simulink model "IMU_UKF_circle_exp_sampling_rate_issue"  (R2025a)
settings: Solver=FixedStepAuto  StartTime=0.0  StopTime=inf  FixedStep=0.01  RelTol=1e-3
undefined symbols (not defined in the file or in its folder): National_Instruments, PCI
libraries: sldrtlib x3, slpidlib x2, hostiolib x1
settings Model: Creator=dperera  LastModifiedBy=dperera

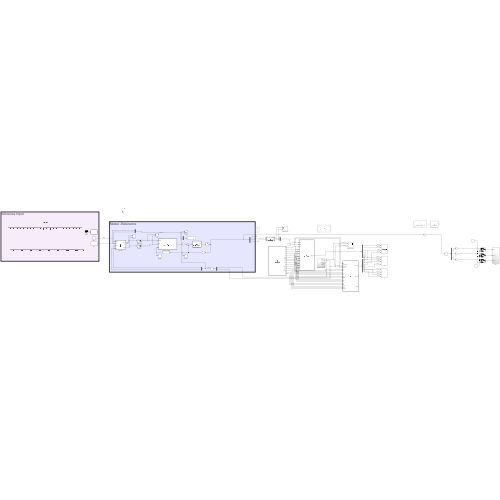
[thumbnail: Simulink's stored preview of the top-level diagram]
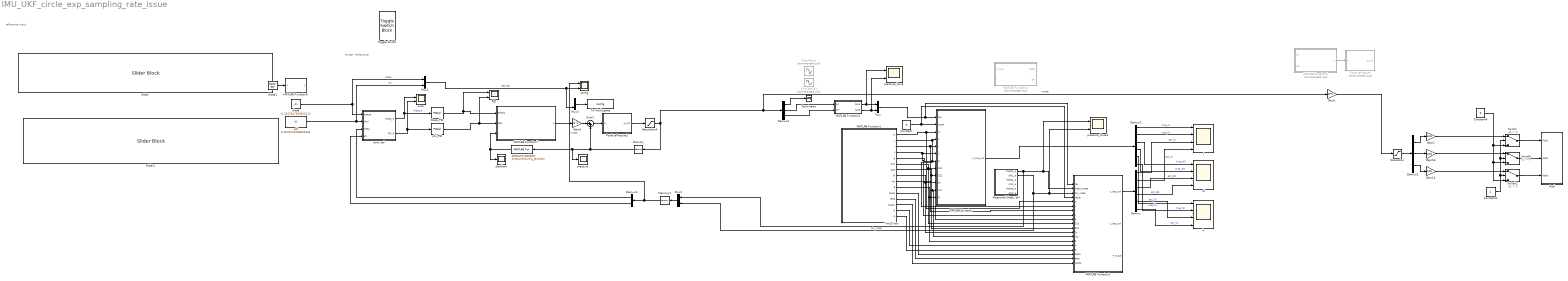
== system IMU_UKF_circle_exp_sampling_rate_issue ==
  note: reference Input
  note: Model -Reference
  Constant : Constant  Value=0
  Constant1 : Constant
  Constant4 : Constant  Value=0
  Demux : Demux  Outputs=6
  Demux1 : Demux  Outputs=6
  Demux2 : Demux  Outputs=3
  Demux3 : Demux  Outputs=2
  Demux4 : Demux  Outputs=3
  Gain1 : Gain  Gain=1e-5
  Gain14 : Gain  Gain=10/9
  Gain16 : Gain  Gain=10/9
  Gain2 : Gain  Gain=10/9
  Gain3 : Gain  Gain=0.1
  Jacobian : Scope
      settings: ActiveDisplayYMinimum=-10.825317547305481  ActiveDisplayYMaximum=10.825317547305481  DataLoggingVariableName=ScopeData5
  MATLAB Function : MATLAB Function  TreatAsAtomicUnit=on
  MATLAB Function1 : MATLAB Function  TreatAsAtomicUnit=on
  MATLAB Function2 : MATLAB Function  Commented=on  TreatAsAtomicUnit=on
  MATLAB Function3 : MATLAB Function  TreatAsAtomicUnit=on
  MATLAB Function4 : MATLAB Function  TreatAsAtomicUnit=on
  MATLAB Function5 : MATLAB Function  Commented=on  TreatAsAtomicUnit=on
  MATLAB Function6 : MATLAB Function  TreatAsAtomicUnit=on
  MATLAB Function7 : MATLAB Function  TreatAsAtomicUnit=on
  "Measured theta, phi" : Subsystem
  Memory : Memory  InitialCondition=[1; 1.1; 1]  LinearizeMemory=on  LinearizeAsDelay=on
  Memory1 : Memory  InitialCondition=[0.0001, 0.0001]  LinearizeMemory=on  LinearizeAsDelay=on
  Mux{,1..3} (4 alike) : Mux  Inputs=2
  PID : Scope  NumInputPorts=2
      settings: ActiveDisplayYMinimum=-3.9804584732791981  ActiveDisplayYMaximum=3.8453740981888478  DataLoggingVariableName=ScopeData6
  PositivePresure : MATLAB Function  Commented=on  TreatAsAtomicUnit=on
  PositivePresure1 : MATLAB Function  TreatAsAtomicUnit=on
  "Red " : Subsystem
  Saturation : Saturate  UpperLimit=3  LowerLimit=0
  Saturation4 : Saturate  UpperLimit=300000  LowerLimit=0
  Sine Wave : Sin  Commented=on  Amplitude=2.5e4  Frequency=0.5  SampleTime=0
  Sine Wave1 : Sin  Commented=on  Amplitude=2.5e4  Frequency=0.5  SampleTime=0
  Slider : SliderBlock  ScaleMin=-3.14  ScaleMax=3.14
  Slider1 : SliderBlock  ScaleMax=3.14
  Sum2 : Sum  Inputs=|++
  Switch : Switch  Criteria=u2 > Threshold  SaturateOnIntegerOverflow=off  InputSameDT=off
  Switch1 : Switch  Criteria=u2 > Threshold  SaturateOnIntegerOverflow=off  InputSameDT=off
  Switch2 : Switch  Criteria=u2 > Threshold  SaturateOnIntegerOverflow=off  InputSameDT=off
  Terminator : Terminator
  To Workspace : ToWorkspace  VariableName=config  SaveFormat=Structure With Time  SampleTime=-1
  Toggle Switch : ToggleSwitchBlock
  config : Scope  NumInputPorts=2
      settings: ActiveDisplayYMinimum=-3.926205418823844  ActiveDisplayYMaximum=3.9199222335166648  DataLoggingVariableName=ScopeData7
  dl : Scope  NumInputPorts=4
      settings: ActiveDisplayYMinimum=-0.11562375107326617  ActiveDisplayYMaximum=0.16522740194349217
  error : Scope  NumInputPorts=2
      settings: ActiveDisplayYMinimum=-1.7062614665873941  ActiveDisplayYMaximum=3.7647403361072445  DataLoggingVariableName=ScopeData9
  error cal : MATLAB Function  TreatAsAtomicUnit=on
  h : Scope  NumInputPorts=4
      settings: ActiveDisplayYMinimum=-3.6910086116177509E-9  ActiveDisplayYMaximum=1.6868676985022998E-9  DataLoggingVariableName=ScopeData2
  l : Scope  NumInputPorts=4
      settings: ActiveDisplayYMinimum=-0.05861032867923114  ActiveDisplayYMaximum=0.027492958113080231
  phi : Constant  Value=0.4033234086825366
  phi_PID : slpidlib/PID Controller  Controller=PID  Form=Parallel  TimeDomain=Continuous-time  UseExternalTs=off  SampleTime=-1  IntegratorMethod=Forward Euler  FilterMethod=Forward Euler  ControllerParametersSource=internal  P=0.1  I=0.01  UseKiTs=off  D=0.00001  UseExternalDerivativeSource=off  N=100  UseFilter=on  TunerSelectOption=Transfer Function Based (PID Tuner App)  InitialConditionSource=internal  InitialConditionForIntegrator=0  InitialConditionForFilter=0  DifferentiatorICPrevScaledInput=0  ExternalReset=none  TrackingMode=off  Kt=1  LimitOutput=on  SatLimitsSource=internal  UpperSaturationLimit=inf  LowerSaturationLimit=-inf  LinearizeAsGain=off  AntiWindupMode=back-calculation  Kb=1  LimitIntegrator=off  UpperIntegratorSaturationLimit=10  LowerIntegratorSaturationLimit=-10  POutMin=[]  POutMax=[]  IOutMin=[]  IOutMax=[]  DOutMin=[]  DOutMax=[]  NOutMin=[]  NOutMax=[]  SumOutMin=[]  SumOutMax=[]  SaturationOutMin=[]  SaturationOutMax=[]  PParamMin=[]  PParamMax=[]  IParamMin=[]  IParamMax=[]  DParamMin=[]  DParamMax=[]  NParamMin=[]  NParamMax=[]  KbParamMin=[]  KbParamMax=[]  KtParamMin=[]  KtParamMax=[]  KbOutMin=[]  KbOutMax=[]  KtOutMin=[]  KtOutMax=[]  IntegratorOutMin=[]  IntegratorOutMax=[]  FilterOutMin=[]  FilterOutMax=[]  SumI1OutMin=[]  SumI1OutMax=[]  SumI2OutMin=[]  SumI2OutMax=[]  SumI3OutMin=[]  SumI3OutMax=[]  SumI4OutMin=[]  SumI4OutMax=[]  SumDOutMin=[]  SumDOutMax=[]  DifferentiatorOutMin=[]  DifferentiatorOutMax=[]  FilterDiffOutCoefMin=[]  FilterDiffOutCoefMax=[]  ReciprocalOutMin=[]  ReciprocalOutMax=[]  SumDenOutMin=[]  SumDenOutMax=[]  SumNumOutMin=[]  SumNumOutMax=[]  DivideOutMin=[]  DivideOutMax=[]  UdiffTsProdOutMin=[]  UdiffTsProdOutMax=[]  NTsProdOutMin=[]  NTsProdOutMax=[]  UintegralTsProdOutMin=[]  UintegralTsProdOutMax=[]  UngainTsProdOutMin=[]  UngainTsProdOutMax=[]  ClampingZeroOutDataTypeStr=Inherit: Inherit via back propagation  ClampingZeroOutMin=[]  ClampingZeroOutMax=[]  FilterDenConstantOutDataTypeStr=Inherit: Inherit via back propagation  FilterDenConstantOutMin=[]  FilterDenConstantOutMax=[]  PCopyOutDataTypeStr=Inherit: Inherit via back propagation  PCopyOutMin=[]  PCopyOutMax=[]  NCopyOutDataTypeStr=Inherit: Inherit via back propagation  NCopyOutMin=[]  NCopyOutMax=[]  IntegratorContinuousStateAttributes=''  IntegratorStateMustResolveToSignalObject=off  IntegratorRTWStateStorageClass=Auto  FilterContinuousStateAttributes=''  FilterStateMustResolveToSignalObject=off  FilterRTWStateStorageClass=Auto  ParallelPVariant=InternalParameters  IdealPVariant=Disabled  IVariant=InternalParameters  DVariant=InternalParameters  IntegratorVariant=Continuous  SatVariant=Enabled  AWVariant=BackCalculation  PCopyVariant=Disabled  TRVariant=Disabled  FdbkBlocksVariant=Forward  IdealPFdbkVariant=Disabled  SatFdbkVariant=Disabled  DerivativeFilterVariant=ContFilter  NVariant=InternalParameters  NCopyVariant=Disabled  FilterICVariant=InternalICsFilter  IntegratorICVariant=InternalICs  ExternalResetVariant=Disabled  TRSumVariant=Passthrough  SumFdbkVariant=Disabled  SumVariant=Sum_PID  TsampFilterVariant=InternalTs  TsampNgainVariant=Passthrough  TsampIntegralVariant=Disabled_SignalSpec  ExternalSaturationOutDataTypeStr=Inherit: Same as second input  DerivativeSourceVariant=ErrorSignal  PreIntVariant=InternalPreInt
  pressure : Scope
      settings: ActiveDisplayYMinimum=-37499.999999999993  ActiveDisplayYMaximum=337500  DataLoggingVariableName=ScopeData10
  pressure_force : Scope  NumInputPorts=2
      settings: ActiveDisplayYMinimum=-1  ActiveDisplayYMaximum=1  DataLoggingVariableName=ScopeData3
  pressure_force1 : Scope  NumInputPorts=2
      settings: ActiveDisplayYMinimum=-0.05267150170136882  ActiveDisplayYMaximum=1.3490874232227761  DataLoggingVariableName=ScopeData4
  pressure_jacobian : MATLABFcn  MATLABFcn=pressure2config_Jacobian  OutputDimensions=[2 3]  OutputSignalType=real  Output1D=off
  theta : Constant  Value=-0.2347847506630112
  theta1 : SignalGenerator  WaveForm=sawtooth  Amplitude=pi  Frequency=0.2*2*pi  Units=rad/sec  VectorParams1D=off
  theta_PID : slpidlib/PID Controller  Controller=PID  Form=Parallel  TimeDomain=Continuous-time  UseExternalTs=off  SampleTime=-1  IntegratorMethod=Forward Euler  FilterMethod=Forward Euler  ControllerParametersSource=internal  P=0.1  I=0.01  UseKiTs=off  D=0.0001  UseExternalDerivativeSource=off  N=100  UseFilter=on  TunerSelectOption=Transfer Function Based (PID Tuner App)  InitialConditionSource=internal  InitialConditionForIntegrator=0  InitialConditionForFilter=0  DifferentiatorICPrevScaledInput=0  ExternalReset=none  TrackingMode=off  Kt=1  LimitOutput=on  SatLimitsSource=internal  UpperSaturationLimit=inf  LowerSaturationLimit=-inf  LinearizeAsGain=off  AntiWindupMode=back-calculation  Kb=1  LimitIntegrator=off  UpperIntegratorSaturationLimit=10  LowerIntegratorSaturationLimit=-10  POutMin=[]  POutMax=[]  IOutMin=[]  IOutMax=[]  DOutMin=[]  DOutMax=[]  NOutMin=[]  NOutMax=[]  SumOutMin=[]  SumOutMax=[]  SaturationOutMin=[]  SaturationOutMax=[]  PParamMin=[]  PParamMax=[]  IParamMin=[]  IParamMax=[]  DParamMin=[]  DParamMax=[]  NParamMin=[]  NParamMax=[]  KbParamMin=[]  KbParamMax=[]  KtParamMin=[]  KtParamMax=[]  KbOutMin=[]  KbOutMax=[]  KtOutMin=[]  KtOutMax=[]  IntegratorOutMin=[]  IntegratorOutMax=[]  FilterOutMin=[]  FilterOutMax=[]  SumI1OutMin=[]  SumI1OutMax=[]  SumI2OutMin=[]  SumI2OutMax=[]  SumI3OutMin=[]  SumI3OutMax=[]  SumI4OutMin=[]  SumI4OutMax=[]  SumDOutMin=[]  SumDOutMax=[]  DifferentiatorOutMin=[]  DifferentiatorOutMax=[]  FilterDiffOutCoefMin=[]  FilterDiffOutCoefMax=[]  ReciprocalOutMin=[]  ReciprocalOutMax=[]  SumDenOutMin=[]  SumDenOutMax=[]  SumNumOutMin=[]  SumNumOutMax=[]  DivideOutMin=[]  DivideOutMax=[]  UdiffTsProdOutMin=[]  UdiffTsProdOutMax=[]  NTsProdOutMin=[]  NTsProdOutMax=[]  UintegralTsProdOutMin=[]  UintegralTsProdOutMax=[]  UngainTsProdOutMin=[]  UngainTsProdOutMax=[]  ClampingZeroOutDataTypeStr=Inherit: Inherit via back propagation  ClampingZeroOutMin=[]  ClampingZeroOutMax=[]  FilterDenConstantOutDataTypeStr=Inherit: Inherit via back propagation  FilterDenConstantOutMin=[]  FilterDenConstantOutMax=[]  PCopyOutDataTypeStr=Inherit: Inherit via back propagation  PCopyOutMin=[]  PCopyOutMax=[]  NCopyOutDataTypeStr=Inherit: Inherit via back propagation  NCopyOutMin=[]  NCopyOutMax=[]  IntegratorContinuousStateAttributes=''  IntegratorStateMustResolveToSignalObject=off  IntegratorRTWStateStorageClass=Auto  FilterContinuousStateAttributes=''  FilterStateMustResolveToSignalObject=off  FilterRTWStateStorageClass=Auto  ParallelPVariant=InternalParameters  IdealPVariant=Disabled  IVariant=InternalParameters  DVariant=InternalParameters  IntegratorVariant=Continuous  SatVariant=Enabled  AWVariant=BackCalculation  PCopyVariant=Disabled  TRVariant=Disabled  FdbkBlocksVariant=Forward  IdealPFdbkVariant=Disabled  SatFdbkVariant=Disabled  DerivativeFilterVariant=ContFilter  NVariant=InternalParameters  NCopyVariant=Disabled  FilterICVariant=InternalICsFilter  IntegratorICVariant=InternalICs  ExternalResetVariant=Disabled  TRSumVariant=Passthrough  SumFdbkVariant=Disabled  SumVariant=Sum_PID  TsampFilterVariant=InternalTs  TsampNgainVariant=Passthrough  TsampIntegralVariant=Disabled_SignalSpec  ExternalSaturationOutDataTypeStr=Inherit: Same as second input  DerivativeSourceVariant=ErrorSignal  PreIntVariant=InternalPreInt
  wires:
  MATLAB Function1/1(m) -> MATLAB Function3/5(m), MATLAB Function/3(m)
  MATLAB Function1/2(L) -> MATLAB Function/4(L), MATLAB Function3/6(L)
  MATLAB Function1/3(r) -> MATLAB Function3/7(r), MATLAB Function/5(r)
  MATLAB Function1/4(k) -> MATLAB Function3/8(k), MATLAB Function/6(k)
  MATLAB Function1/5(g) -> MATLAB Function3/9(g), MATLAB Function/7(g)
  MATLAB Function1/6(D11) -> MATLAB Function3/10(D11), MATLAB Function/8(D11)
  MATLAB Function1/7(D22) -> MATLAB Function3/11(D22), MATLAB Function/9(D22)
  MATLAB Function1/8(Ts) -> MATLAB Function3/12(Ts), MATLAB Function/10(Ts)
  MATLAB Function1/9(rho) -> MATLAB Function3/13(rho), MATLAB Function/11(rho)
  MATLAB Function1/10(B) -> MATLAB Function3/14(B), MATLAB Function/12(B)
  MATLAB Function/1(x_true_out) -> Demux1/1
  MATLAB Function1/11(alpha) -> MATLAB Function3/17(alpha)
  MATLAB Function1/12(beta) -> MATLAB Function3/18(beta)
  MATLAB Function1/13(kappa) -> MATLAB Function3/19(kappa)
  MATLAB Function1/14(Q) -> MATLAB Function3/15(Q)
  MATLAB Function1/15(R) -> MATLAB Function3/16(R)
  Constant/1 -> MATLAB Function3/4(reset), MATLAB Function/2(reset)
  Mux/1 -> MATLAB Function3/1(tau), MATLAB Function/1(tau)
  MATLAB Function3/1(x_hat_out) -> Demux/1
  Demux1/1 -> l/1  "true_l2"
  Demux/1 -> l/3  "est_l2"
  Demux1/2 -> l/2  "true_l3"
  Demux/2 -> l/4  "est_l3"
  Demux1/3 -> dl/1  "true_dl2"
  Demux1/4 -> dl/2  "true_dl3"
  Demux/3 -> dl/3  "est_dl2"
  Demux/4 -> dl/4  "est_dl3"
  Demux1/5 -> h/1  "true_h1"
  Demux1/6 -> h/2  "true_h2"
  Demux/5 -> h/3  "est_h1"
  Demux/6 -> h/4  "est_h2"
  MATLAB Function4/1(tau2) -> pressure_force/1, Mux/1
  MATLAB Function4/2(tau3) -> Mux/2, pressure_force/2
  Demux4/2 -> MATLAB Function4/1(p2)
  Demux4/3 -> MATLAB Function4/2(p3)
  "Measured theta, phi"/1(theta1_a) -> Mux2/1, pressure_force1/1, MATLAB Function3/2(theta_meas)  "theta_meas"
  "Measured theta, phi"/2(phi1_a) -> Mux2/2, pressure_force1/2, MATLAB Function3/3(phi_meas)  "phi_meas"
  Demux2/2 -> Gain16/1
  Demux2/3 -> Gain14/1
  Switch2/1 -> "Red "/3(Red3)
  Constant4/1 -> Switch2/3, Switch1/3, Switch/3
  Demux2/1 -> Gain2/1
  Gain16/1 -> Switch1/1
  Gain2/1 -> Switch/1
  Switch1/1 -> "Red "/2(Red2)
  Switch/1 -> "Red "/1(Red1)
  MATLAB Function5/1(p) -> PositivePresure/1(p)
  Gain14/1 -> Switch2/1
  Saturation/1 -> Demux2/1
  Constant1/1 -> Switch2/2, Switch1/2, Switch/2
  Mux3/1 -> To Workspace/1
  error cal/2(phi_e) -> error/2, phi_PID/1
  Mux1/1 -> config/2, Mux3/2  "desired"
  theta/1 -> Mux1/1, error cal/1(thetad)  "theta"
  phi/1 -> Mux1/2, error cal/2(phid)  "phi"
  Sum2/1 -> PositivePresure1/1(p)
  phi_PID/1 -> PID/2, MATLAB Function7/2(dphi)
  Demux3/2 -> error cal/4(phi)
  theta1/1 -> MATLAB Function6/1(u)
  PositivePresure1/1(p_out) -> Saturation4/1
  Gain3/1 -> Sum2/1
  Memory1/1 -> config/1, Demux3/1  "model"
  pressure_jacobian/1 -> Jacobian/1, MATLAB Function7/3(J)
  MATLAB Function7/1(p) -> Gain3/1
  Memory/1 -> pressure/1, pressure_jacobian/1, Sum2/2
  Saturation4/1 -> Gain1/1, Demux4/1, Memory/1  "model"
  Demux3/1 -> error cal/3(theta)
  error cal/1(theta_e) -> error/1, theta_PID/1  "theta_e"
  theta_PID/1 -> PID/1, MATLAB Function7/1(dtheta)
  Mux2/1 -> Memory1/1
  Gain1/1 -> Saturation/1
  Demux4/1 -> Terminator/1

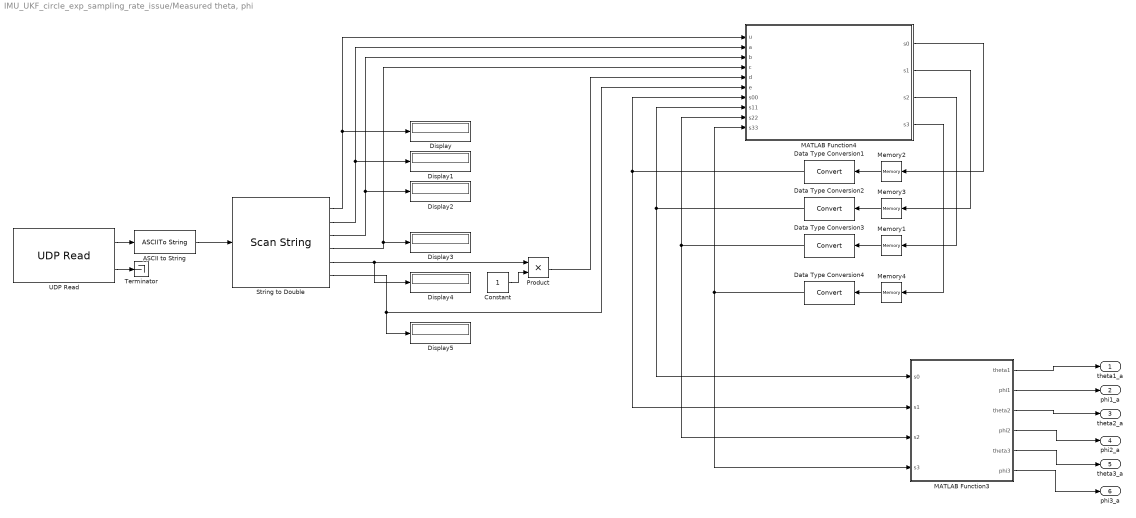
== system IMU_UKF_circle_exp_sampling_rate_issue/Measured theta, phi ==
  ASCII to String : ASCIIToString
  Constant : Constant
  Data Type Conversion{1..4} (4 alike) : DataTypeConversion  SaturateOnIntegerOverflow=off  RndMeth=Floor
  Display{,1..5} (6 alike) : Display
  MATLAB Function3 : MATLAB Function  TreatAsAtomicUnit=on
  MATLAB Function4 : MATLAB Function  TreatAsAtomicUnit=on
  Memory1 : Memory  InitialCondition=[1.0,0,0,0,0,1]  InheritSampleTime=on
  Memory2 : Memory  InitialCondition=[0.0,0,0,0,0,1]  InheritSampleTime=on
  Memory3 : Memory  InitialCondition=[1.0,0,0,0,0,1]  InheritSampleTime=on
  Memory4 : Memory  InitialCondition=[1.0,0,0,0,0,1]  InheritSampleTime=on
  Product : Product
  String to Double : ScanString  Format="\"%f %f %f %f %f %f\""
  Terminator : Terminator
  UDP Read : hostiolib/UDP Read  localURL='0.0.0.0'  localPort=60002  remoteURL='localhost'  remotePort=-1  recvBufferSize=1024  dims=255  signalDatatype=uint8  isVarSize=off  showBlockingTime=on  blockingTime=0  sampletime=0.01  blockPlatform=HOST  hoistedMaskSrc=UDP Read/UDP Read Sim/UDP Read
  theta1_a : Outport
  phi1_a : Outport  Port=2
  theta2_a : Outport  Port=3
  phi2_a : Outport  Port=4
  theta3_a : Outport  Port=5
  phi3_a : Outport  Port=6
  wires:
  ASCII to String/1 -> String to Double/1
  Memory4/1 -> Data Type Conversion4/1
  Constant/1 -> Product/2
  UDP Read/2 -> Terminator/1
  UDP Read/1 -> ASCII to String/1
  String to Double/2 -> MATLAB Function4/2(a), Display1/1
  String to Double/1 -> Display/1, MATLAB Function4/1(u)
  MATLAB Function4/3(s2) -> Memory1/1
  Data Type Conversion4/1 -> MATLAB Function3/4(s3), MATLAB Function4/10(s33)
  String to Double/6 -> Display5/1, MATLAB Function4/6(e)
  Product/1 -> MATLAB Function4/5(d)
  String to Double/4 -> MATLAB Function4/4(c), Display3/1
  String to Double/5 -> Display4/1, Product/1
  Memory2/1 -> Data Type Conversion1/1
  Data Type Conversion2/1 -> MATLAB Function3/1(s0), MATLAB Function4/8(s11)
  Memory1/1 -> Data Type Conversion3/1
  MATLAB Function4/4(s3) -> Memory4/1
  MATLAB Function4/2(s1) -> Memory3/1
  Data Type Conversion3/1 -> MATLAB Function3/3(s2), MATLAB Function4/9(s22)
  Memory3/1 -> Data Type Conversion2/1
  MATLAB Function4/1(s0) -> Memory2/1
  Data Type Conversion1/1 -> MATLAB Function3/2(s1), MATLAB Function4/7(s00)
  String to Double/3 -> MATLAB Function4/3(b), Display2/1
  MATLAB Function3/1(theta1) -> theta1_a/1
  MATLAB Function3/2(phi1) -> phi1_a/1
  MATLAB Function3/3(theta2) -> theta2_a/1
  MATLAB Function3/4(phi2) -> phi2_a/1
  MATLAB Function3/5(theta3) -> theta3_a/1
  MATLAB Function3/6(phi3) -> phi3_a/1

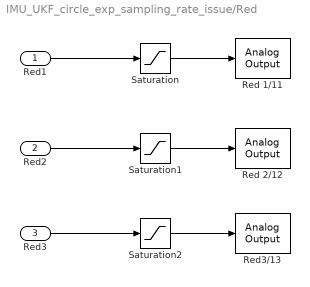
== system IMU_UKF_circle_exp_sampling_rate_issue/Red  ==
  Red1 : Inport
  Red2 : Inport  Port=2
  Red3 : Inport  Port=3
  Red 1/11 : sldrtlib/Analog Output  SampleTime=0.01  MaxMissedTicks=inf  ShowMissedTicks=off  YieldWhenWaiting=on  DrvName=National_Instruments/PCI-6703  DrvAddress=4294967295  DrvOptions=0  Channels=1  RangeMode=1  VoltRange=1  InitialValue=0  FinalValue=0
      settings: AttributesFormatString=National Instruments\nPCI-6703 [auto]
  Red 2/12 : sldrtlib/Analog Output  SampleTime=0.01  MaxMissedTicks=inf  ShowMissedTicks=off  YieldWhenWaiting=on  DrvName=National_Instruments/PCI-6703  DrvAddress=4294967295  DrvOptions=0  Channels=2  RangeMode=1  VoltRange=1  InitialValue=0  FinalValue=0
      settings: AttributesFormatString=National Instruments\nPCI-6703 [auto]
  Red3/13 : sldrtlib/Analog Output  SampleTime=0.01  MaxMissedTicks=inf  ShowMissedTicks=off  YieldWhenWaiting=on  DrvName=National_Instruments/PCI-6703  DrvAddress=4294967295  DrvOptions=0  Channels=3  RangeMode=1  VoltRange=1  InitialValue=0  FinalValue=0
      settings: AttributesFormatString=National Instruments\nPCI-6703 [auto]
  Saturation : Saturate  UpperLimit=7  LowerLimit=0
  Saturation1 : Saturate  UpperLimit=7  LowerLimit=0
  Saturation2 : Saturate  UpperLimit=7  LowerLimit=0
  wires:
  Red1/1 -> Saturation/1
  Saturation/1 -> Red 1/11/1
  Saturation1/1 -> Red 2/12/1
  Saturation2/1 -> Red3/13/1
  Red2/1 -> Saturation1/1
  Red3/1 -> Saturation2/1

== matlab function IMU_UKF_circle_exp_sampling_rate_issue/MATLAB Function4 ==
  data: tau2 output; tau3 output; p2 input; p3 input
function [tau2,tau3] = pressures(p2, p3)
%#codegen

A = pi * (0.013/2)^2;
tau2 = p2*A;
tau3 = p3*A;

end

== matlab function IMU_UKF_circle_exp_sampling_rate_issue/Measured theta, phi/MATLAB Function3 ==
  data: s0 input; theta1 output; s1 input; phi1 output; s2 input; s3 input; theta2 output; phi2 output; theta3 output; phi3 output
function [theta1,phi1,theta2,phi2,theta3,phi3]= fcn(s0,s1,s2,s3)

s0_start=[0,0,0,1];
s1_start=[0,0,0,1];
s2_start=[0,0,0,1];
s3_start=[0,0,0,1];


%base=[base1(3),base1(4),base1(5),base1(6)];

sensor0=[s0(6),s0(3),s0(5),s0(4)]; %base
sensor1=[s1(6),s1(3),s1(5),s1(4)];
sensor2=[s2(6),s2(3),s2(5),s2(4)];
sensor3=[s3(6),s3(3),s3(5),s3(4)];

%tip_relative_base=quatmultiply(quatmultiply(tip,quatinv(tip_start)),quatinv(quatmultiply(base,quatinv(base_start))));

sensor1_relative_sensor0=quatmultiply(quatmultiply(sensor1,quatinv(s1_start)),quatinv(quatmultiply(sensor0,quatinv(s0_start))));
sensor2_relative_sensor1=quatmultiply(quatmultiply(sensor2,quatinv(s2_start)),quatinv(quatmultiply(sensor1,quatinv(s1_start))));
sensor3_relative_sensor2=quatmultiply(quatmultiply(sensor3,quatinv(s3_start)),quatinv(quatmultiply(sensor2,quatinv(s2_start))));

%rotMat = quat2tform(tip_relative_base);
rotMat1 = quat2tform(sensor1_relative_sensor0); % only base
theta1= (atan2(rotMat1(2,3),rotMat1(1,3)));
phi1= (acos(rotMat1(3,3)));

rotMat2 = quat2tform(sensor2_relative_sensor1); 
theta2=  (atan2(rotMat2(2,3),rotMat2(1,3)));
phi2= (acos(rotMat2(3,3)));

rotMat3 = quat2tform(sensor3_relative_sensor2); 
theta3= (atan2(rotMat3(2,3),rotMat3(1,3)));
phi3= (acos(rotMat3(3,3)));


end

== matlab function IMU_UKF_circle_exp_sampling_rate_issue/Measured theta, phi/MATLAB Function4 ==
  data: u input; s0 output; a input; b input; c input; d input; e input; s00 input; s11 input; s1 output; s22 input; s33 input; s2 output; s3 output
function [s0,s1,s2,s3]= fcn(u,a,b,c,d,e,s00,s11,s22,s33)
if u==1.0
    %base1=[double(u),double(a),double(b),double(c),double(d),double(e)];
    s00(1)=double(u);
    s00(2)=double(a);
    s00(3)=double(b); %x
    s00(4)=double(c); %y
    s00(5)=double(d); %z
    s00(6)=double(e); %w

elseif u==2.0
    %tip1=[double(u),double(a),double(b),double(c),double(d),double(e)];
    s11(1)=double(u);
    s11(2)=double(a);
    s11(3)=double(b);
    s11(4)=double(c);
    s11(5)=double(d);
    s11(6)=double(e);
elseif u==3.0
    %tip1=[double(u),double(a),double(b),double(c),double(d),double(e)];
    s22(1)=double(u);
    s22(2)=double(a);
    s22(3)=double(b);
    s22(4)=double(c);
    s22(5)=double(d);
    s22(6)=double(e);
elseif u==4.0
    %tip1=[double(u),double(a),double(b),double(c),double(d),double(e)];
    s33(1)=double(u);
    s33(2)=double(a);
    s33(3)=double(b);
    s33(4)=double(c);
    s33(5)=double(d);
    s33(6)=double(e);
end
    s0=s00;
    s1=s11;
    s2=s22;
    s3=s33;

end

== matlab function IMU_UKF_circle_exp_sampling_rate_issue/MATLAB Function5 ==
  data: p2 input; p output; p3 input
function p = Measurement_Block(p2, p3)
%#codegen

p = [-(p2+p3); p2; p3];

end

== matlab function IMU_UKF_circle_exp_sampling_rate_issue/PositivePresure ==
  data: p input; p_out output
function p_out  = PositivePressure(p)

    minP = min(p);
    maxP = max(p);
    
    p_pos = p-minP;
    % p_pos_norm = p_pos / (maxP - minP) * maxP; % Normalize the positive pressures
    
    p_out = p_pos/max(p_pos) * maxP;
    
end

== matlab function IMU_UKF_circle_exp_sampling_rate_issue/MATLAB Function6 ==
  data: u input; y output
function y = fcn(u)

y = wrapToPi(u - pi);

== matlab function IMU_UKF_circle_exp_sampling_rate_issue/MATLAB Function7 ==
  data: dtheta input; p output; dphi input; J input
function p  = config3pressure_projection(dtheta, dphi, J)

    p = J \ [dtheta; dphi];
end

== matlab function IMU_UKF_circle_exp_sampling_rate_issue/PositivePresure1 ==
  data: p input; p_out output
function p_out  = PositivePressure(p)

    minP = min(p);
    maxP = max(p);
    
    p_pos = p-minP;
    % p_pos_norm = p_pos / (maxP - minP) * maxP; % Normalize the positive pressures
    
    p_out = p_pos/max(p_pos) * maxP;
    
end

== matlab function IMU_UKF_circle_exp_sampling_rate_issue/error cal ==
  data: thetad input; theta_e output; phid input; theta input; phi input; phi_e output
function [theta_e, phi_e]    = fcn(thetad, phid, theta, phi)

    % qd = [thetad;phid];
    % q = [theta;phi];
    % 
    % abs_diff = abs(thetad-theta);
    % abs_diff_mod = abs(mod(thetad, 2*pi)-mod(theta, 2*pi));
    % 
    % if abs_diff < abs_diff_mod
    %     error = qd-q;
    % else
    %     error = mod(qd, 2*pi) - mod(q,2*pi);
    % end
    % 
    % if error(1) < 0.0001
    %     error(1) = 0;
    % end
    % 
    % if error(2) < 0.0001
    %     error(2) = 0;
    % end
    % 
    % theta_e = error(1);
    % phi_e = error(2);

        % Compute signed angular differences in (-pi, pi]
    theta_e = atan2(sin(thetad - theta), cos(thetad - theta));
    phi_e   = atan2(sin(phid - phi), cos(phid - phi));

    % Optional: zero small errors
    if abs(theta_e) < 1e-4
        theta_e = 0;
    end
    if abs(phi_e) < 1e-4
        phi_e = 0;
    end

end

== matlab function IMU_UKF_circle_exp_sampling_rate_issue/MATLAB Function1 ==
  data: m output; L output; r output; k output; g output; D11 output; D22 output; Ts output; rho output; B output; alpha output; beta output; kappa output; Q output; R output
function [m, L, r, k, g, D11, D22, Ts, rho, B, alpha, beta, kappa, Q, R] = parameters()
%#codegen

m    = 0.10;
L    = [0.0; 0.278; 0.0];
r    = 0.013;
k    = [0.0; 2.4e3; 2.4e3];
g    = 9.81;
D11  = 100.0;
D22  = 100.0;
rho  = 0.98;
B    = [1.0; 1.0];
Ts = 0.01;

alpha = 1.0;
beta  = 2.0;
kappa = 0.0;

Q = diag([1e-9, 1e-9, 1e-6, 1e-6, 1e-5, 1e-5]);
R = diag([deg2rad(6)^2, deg2rad(6)^2]);

end

== matlab function IMU_UKF_circle_exp_sampling_rate_issue/MATLAB Function ==
  settings: updateMethod=DISCRETE
  data: tau input; x_true_out output; reset input; m input; L input; r input; k input; g input; D11 input; D22 input; Ts input; rho input; B input
function x_true_out = Plant_Block( ...
    tau, reset, ...
    m, L, r, k, g, D11, D22, Ts, rho, B)
%#codegen
% Discrete-time plant block
%
% Inputs:
%   tau   [2x1] : generalized input force
%   reset [1x1] : reset flag
%
% Parameters:
%   m, L, r, k, g, D11, D22, Ts, rho, B
%
% Output:
%   x_true_out [6x1] = [l2; l3; dl2; dl3; h1; h2]

    persistent x_true isInit

    if isempty(isInit)
        x_true = zeros(6,1);
        isInit = true;
    end

    if reset ~= 0
        % choose a small nonzero bend if you want to avoid phi ~ 0 initially
        x_true = zeros(6,1);
        % x_true = [0.005; -0.004; 0; 0; 0; 0];
    end

    % one discrete-time propagation step
    x_true = processModelPlantLocal(x_true, tau, ...
        m, L, r, k, g, D11, D22, Ts, rho, B);

    x_true_out = x_true;
end


% ============================================================
% LOCAL PROCESS MODEL
% ============================================================
function x_next = processModelPlantLocal(x, tau, ...
    m, L, r, k, g, D11, D22, Ts, rho, B)
%#codegen

    % State unpack
    l_x  = x(1:2);
    dl_x = x(3:4);
    h_x  = x(5:6);

    % Reconstruct full length vector used by symbolic dynamics
    l = zeros(3,1);
    l(1) = 0.0;
    l(2) = l_x(1);
    l(3) = l_x(2);

    % Hysteresis gain matrix
    Bh = zeros(2,2);
    Bh(1,1) = B(1);
    Bh(2,2) = B(2);

    % Damping vector
    D = zeros(2,1);
    D(1) = D11 * dl_x(1);
    D(2) = D22 * dl_x(2);

    % Symbolic dynamics
    M = f20251015_2_M_jointspace_MSF(l, m, L, r);
    C = f20251015_3_C_jointspace_MSF(l, m, L, r, dl_x(1), dl_x(2));
    G = f20251015_4_G_and_K_jointspace_MSF(l, m, L, r, k, g);

    rhs = tau - C*dl_x - G - D + Bh*h_x;

    % Numerical regularization
    M = 0.5 * (M + M.');
    M = M + 1e-6 * eye(2);

    ddl = M \ rhs;

    % Discrete-time update
    l_next  = l_x  + Ts*dl_x + 0.5*Ts*Ts*ddl;
    dl_next = dl_x + Ts*ddl;
    h_next  = rho*h_x;

    % Optional saturation for robustness
    l_lim  = 0.05;
    dl_lim = 1.0;
    h_lim  = 20.0;

    l_next(1)  = min(max(l_next(1),  -l_lim),  l_lim);
    l_next(2)  = min(max(l_next(2),  -l_lim),  l_lim);
    dl_next(1) = min(max(dl_next(1), -dl_lim), dl_lim);
    dl_next(2) = min(max(dl_next(2), -dl_lim), dl_lim);
    h_next(1)  = min(max(h_next(1),  -h_lim),  h_lim);
    h_next(2)  = min(max(h_next(2),  -h_lim),  h_lim);

    x_next = zeros(6,1);
    x_next(1:2) = l_next;
    x_next(3:4) = dl_next;
    x_next(5:6) = h_next;
end

== matlab function IMU_UKF_circle_exp_sampling_rate_issue/MATLAB Function2 ==
  data: x_true input; theta output; r input; phi output
function [theta, phi] = Measurement_Block(x_true, r)
%#codegen
% Measurement model block
%
% Inputs:
%   x_true [6x1] : true plant state
%                  [l2; l3; dl2; dl3; h1; h2]
%   r      [1x1] : radial offset
%
% Output:
%   y_meas [2x1] : [theta; phi]

    % State extraction
    l_x = zeros(2,1);
    l_x(1) = x_true(1);
    l_x(2) = x_true(2);

    % Reconstruct full length vector used in CC model
    l = zeros(3,1);
    l(1) = 0.0;
    l(2) = l_x(1);
    l(3) = l_x(2);

    % Bending direction
    theta = atan2(l(3) - l(2), sqrt(3.0) * (l(2) + l(3)));
    theta = wrapAngleLocal(theta);

    % Bending magnitude
    phi = (2.0 / (3.0 * r)) * sqrt( ...
        3.0 * l(2) * l(2) + ...
        3.0 * l(3) * l(2) + ...
        3.0 * l(3) * l(3));

    if phi < 0.0
        phi = 0.0;
    end

end


% ============================================================
% LOCAL ANGLE WRAP
% ============================================================
function a = wrapAngleLocal(a)
%#codegen
    a = mod(a + pi, 2.0*pi) - pi;
end

== matlab function IMU_UKF_circle_exp_sampling_rate_issue/MATLAB Function3 ==
  settings: updateMethod=DISCRETE
  data: tau input; theta_meas input; phi_meas input; x_hat_out output; reset input; m input; L input; r input; k input; g input; D11 input; D22 input; Ts input; rho input; B input; Q input; R input; alpha input; beta input; kappa input; y_hat_out output; P_trace output
function [x_hat_out, y_hat_out, P_trace] = UKF_Block( ...
    tau, theta_meas, phi_meas, reset, ...
    m, L, r, k, g, D11, D22, Ts, rho, B, Q, R, alpha, beta, kappa)
%#codegen
% UKF estimator block
%
% Inputs:
%   tau        [2x1] : generalized input force
%   theta_meas [1x1] : measured theta
%   phi_meas   [1x1] : measured phi
%   reset      [1x1] : reset flag
%
% Parameters:
%   m, L, r, k, g, D11, D22, Ts, rho, B, Q, R, alpha, beta, kappa
%
% Outputs:
%   x_hat_out  [6x1] : estimated state [l2; l3; dl2; dl3; h1; h2]
%   y_hat_out  [2x1] : predicted measurement [theta; phi]
%   P_trace    [1x1] : trace of covariance

    persistent x_hat P isInit

    if isempty(isInit)
        x_hat = zeros(6,1);
        P = diag([1e-5, 1e-5, 1e-4, 1e-4, 1e-3, 1e-3]);
        isInit = true;
    end

    if reset ~= 0
        x_hat = zeros(6,1);
        P = diag([1e-5, 1e-5, 1e-4, 1e-4, 1e-3, 1e-3]);
    end

    % Measurement vector
    y_meas = zeros(2,1);
    y_meas(1) = theta_meas;
    y_meas(2) = phi_meas;

    % Pack process-model input
    u_proc = zeros(23,1);
    u_proc(1:6)   = x_hat;   % placeholder, overwritten for each sigma point
    u_proc(7:8)   = tau;
    u_proc(9)     = m;
    u_proc(10:12) = L;
    u_proc(13)    = r;
    u_proc(14:16) = k;
    u_proc(17)    = g;
    u_proc(18)    = D11;
    u_proc(19)    = D22;
    u_proc(20)    = Ts;
    u_proc(21)    = rho;
    u_proc(22:23) = B;

    % One UKF step
    [x_hat, P, y_hat] = ukfStepLocal( ...
        x_hat, P, u_proc, y_meas, r, Q, R, alpha, beta, kappa);

    x_hat_out = x_hat;
    y_hat_out = y_hat;
    P_trace   = trace(P);
end


% ============================================================
% UKF STEP
% ============================================================
function [x_hat, P, y_pred] = ukfStepLocal( ...
    x_hat, P, u_proc, y_meas, r, Q, R, alpha, beta, kappa)
%#codegen

    [x_pred, P_pred, X_pred, Wm, Wc] = ukfPredictLocal( ...
        x_hat, P, u_proc, Q, alpha, beta, kappa);

    [x_hat, P, y_pred] = ukfUpdateLocal( ...
        x_pred, P_pred, X_pred, y_meas, r, R, Wm, Wc);

    P = 0.5 * (P + P.');
    P = P + 1e-10 * eye(6);
end


% ============================================================
% UKF PREDICT
% ============================================================
function [x_pred, P_pred, X_pred, Wm, Wc] = ukfPredictLocal( ...
    x, P, u_proc, Q, alpha, beta, kappa)
%#codegen

    nx = 6;
    nSigma = 2*nx + 1;

    [X, Wm, Wc] = sigmaPointsLocal(x, P, alpha, beta, kappa);

    X_pred = zeros(nx, nSigma);
    u_i = zeros(23,1);

    for i = 1:nSigma
        u_i = u_proc;
        u_i(1:6) = X(:,i);
        X_pred(:,i) = processModelLocal(u_i);
    end

    x_pred = zeros(nx,1);
    for i = 1:nSigma
        x_pred = x_pred + Wm(i) * X_pred(:,i);
    end

    P_pred = zeros(nx,nx);
    for i = 1:nSigma
        dx = X_pred(:,i) - x_pred;
        P_pred = P_pred + Wc(i) * (dx * dx.');
    end

    P_pred = P_pred + Q;
    P_pred = 0.5 * (P_pred + P_pred.');
    P_pred = P_pred + 1e-10 * eye(nx);
end


% ============================================================
% UKF UPDATE
% ============================================================
function [x_upd, P_upd, y_pred] = ukfUpdateLocal( ...
    x_pred, P_pred, X_pred, y_meas, r, R, Wm, Wc)
%#codegen

    nx = 6;
    ny = 2;
    nSigma = 13;

    Y = zeros(ny, nSigma);
    for i = 1:nSigma
        Y(:,i) = measurementModelLocal(X_pred(:,i), r);
    end

    % Predicted measurement mean
    csum = 0.0;
    ssum = 0.0;
    for i = 1:nSigma
        csum = csum + Wm(i) * cos(Y(1,i));
        ssum = ssum + Wm(i) * sin(Y(1,i));
    end

    y_pred = zeros(2,1);
    y_pred(1) = wrapAngleLocal(atan2(ssum, csum));

    for i = 1:nSigma
        y_pred(2) = y_pred(2) + Wm(i) * Y(2,i);
    end

    % Covariances
    S   = zeros(ny, ny);
    Pxy = zeros(nx, ny);

    for i = 1:nSigma
        dx = X_pred(:,i) - x_pred;

        dy = zeros(ny,1);
        dy(1) = wrapAngleLocal(Y(1,i) - y_pred(1));
        dy(2) = Y(2,i) - y_pred(2);

        S   = S   + Wc(i) * (dy * dy.');
        Pxy = Pxy + Wc(i) * (dx * dy.');
    end

    % Adaptive theta weighting near low curvature
    R_eff = R;
    if y_meas(2) < 0.05
        R_eff(1,1) = 1000.0 * R(1,1);
    end

    S = S + R_eff;
    S = 0.5 * (S + S.');
    S = S + 1e-10 * eye(2);

    K = Pxy / S;

    innov = zeros(ny,1);
    innov(1) = wrapAngleLocal(y_meas(1) - y_pred(1));
    innov(2) = y_meas(2) - y_pred(2);

    x_upd = x_pred + K * innov;

    P_upd = P_pred - K * S * K.';
    P_upd = 0.5 * (P_upd + P_upd.');
    P_upd = P_upd + 1e-10 * eye(nx);
end


% ============================================================
% SIGMA POINTS
% ============================================================
function [X, Wm, Wc] = sigmaPointsLocal(x, P, alpha, beta, kappa)
%#codegen

    nx = 6;
    nSigma = 2*nx + 1;

    lambda = alpha*alpha*(nx + kappa) - nx;
    c = nx + lambda;

    X  = zeros(nx, nSigma);
    Wm = zeros(1, nSigma);
    Wc = zeros(1, nSigma);

    P = 0.5 * (P + P.');
    P = P + 1e-10 * eye(nx);

    S = chol(c * P, 'lower');

    X(:,1) = x;
    for i = 1:nx
        X(:,i+1)    = x + S(:,i);
        X(:,i+1+nx) = x - S(:,i);
    end

    Wm(1) = lambda / c;
    Wc(1) = lambda / c + (1.0 - alpha*alpha + beta);

    for i = 2:nSigma
        Wm(i) = 1.0 / (2.0*c);
        Wc(i) = 1.0 / (2.0*c);
    end
end


% ============================================================
% INTERNAL PROCESS MODEL FOR UKF PREDICTION
% ============================================================
function x_next = processModelLocal(u)
%#codegen

    l_x  = u(1:2);
    dl_x = u(3:4);
    h_x  = u(5:6);
    tau  = u(7:8);
    m    = u(9);
    L    = u(10:12);
    r    = u(13);
    k    = u(14:16);
    g    = u(17);
    D11  = u(18);
    D22  = u(19);
    Ts   = u(20);
    rho  = u(21);
    B    = u(22:23);

    l = zeros(3,1);
    l(1) = 0.0;
    l(2) = l_x(1);
    l(3) = l_x(2);

    Bh = zeros(2,2);
    Bh(1,1) = B(1);
    Bh(2,2) = B(2);

    D = zeros(2,1);
    D(1) = D11 * dl_x(1);
    D(2) = D22 * dl_x(2);

    M = f20251015_2_M_jointspace_MSF(l, m, L, r);
    C = f20251015_3_C_jointspace_MSF(l, m, L, r, dl_x(1), dl_x(2));
    G = f20251015_4_G_and_K_jointspace_MSF(l, m, L, r, k, g);

    rhs = tau - C*dl_x - G - D + Bh*h_x;

    M = 0.5 * (M + M.');
    M = M + 1e-6 * eye(2);

    ddl = M \ rhs;

    l_next  = l_x  + Ts*dl_x + 0.5*Ts*Ts*ddl;
    dl_next = dl_x + Ts*ddl;
    h_next  = rho*h_x;

    % Optional clamping
    l_lim  = 0.05;
    dl_lim = 1.0;
    h_lim  = 20.0;

    l_next(1)  = min(max(l_next(1),  -l_lim),  l_lim);
    l_next(2)  = min(max(l_next(2),  -l_lim),  l_lim);
    dl_next(1) = min(max(dl_next(1), -dl_lim), dl_lim);
    dl_next(2) = min(max(dl_next(2), -dl_lim), dl_lim);
    h_next(1)  = min(max(h_next(1),  -h_lim),  h_lim);
    h_next(2)  = min(max(h_next(2),  -h_lim),  h_lim);

    x_next = zeros(6,1);
    x_next(1:2) = l_next;
    x_next(3:4) = dl_next;
    x_next(5:6) = h_next;
end


% ============================================================
% INTERNAL MEASUREMENT MODEL FOR UKF UPDATE
% ============================================================
function y = measurementModelLocal(x, r)
%#codegen

    l_x = x(1:2);

    l = zeros(3,1);
    l(1) = 0.0;
    l(2) = l_x(1);
    l(3) = l_x(2);

    theta = atan2(l(3) - l(2), sqrt(3.0) * (l(2) + l(3)));
    theta = wrapAngleLocal(theta);

    phi = (2.0 / (3.0 * r)) * sqrt( ...
        3.0*l(2)*l(2) + ...
        3.0*l(3)*l(2) + ...
        3.0*l(3)*l(3));

    if phi < 0.0
        phi = 0.0;
    end

    y = zeros(2,1);
    y(1) = theta;
    y(2) = phi;
end


% ============================================================
% ANGLE WRAP
% ============================================================
function a = wrapAngleLocal(a)
%#codegen
    a = mod(a + pi, 2.0*pi) - pi;
end
